simulink model "CombinatorialLogic"  (Simulink 5.0)
settings: Solver=FixedStepDiscrete  StartTime=0.0  StopTime=10.0  RelTol=1e-3
settings Model: Creator=sofronis  LastModifiedBy=sofronis  ExtModeAutoUpdateStatusClock=off  AlgebraicLoopMsg=error

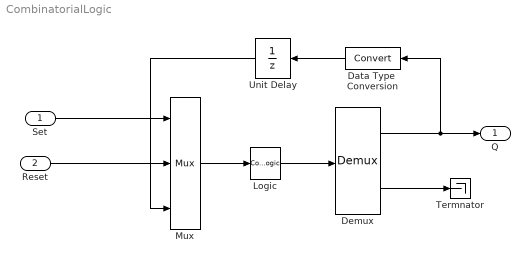
== system CombinatorialLogic ==
  Set : Inport  SampleTime=1  Interpolate=off
  Reset : Inport  Port=2  SampleTime=1
  Data Type  Conversion : DataTypeConversion  Orientation=left  DataType=boolean  SaturateOnIntegerOverflow=on
  Demux : Demux  Outputs=2
  Logic : CombinatorialLogic  TruthTable="[ 0      1;1 1;0 1; 1 1;;;0 0;0.0 1; 0 1; 2.0 0 ]"
  Mux : Mux  Inputs=3
  Termnator : Terminator
  Unit Delay : UnitDelay  Orientation=left
      settings: AttributesFormatString=<initial=%<x0>>\n<tsample=%<sampleTime>>
  Q : Outport
  wires:
  Reset/1 -> Mux/2
  Set/1 -> Mux/1
  Demux/1 -> Q/1, Data Type  Conversion/1
  Demux/2 -> Termnator/1
  Logic/1 -> Demux/1
  Mux/1 -> Logic/1
  Unit Delay/1 -> Mux/3
  Data Type  Conversion/1 -> Unit Delay/1
